simulink model "pharmacokinetics_model"  (R2022b)
settings: Solver=VariableStepAuto  StartTime=0.0  StopTime=total_time  RelTol=1e-3
values from neighbouring files (symbols this model uses):
  alpha = log(2)/half_life_bloodstream    [parameters.m]
  beta = log(2)/half_life_gi_tract    [parameters.m]
  initial_dosage = dosage_amount*60    (= 60000)    [parameters.m]
  pulse_period = 6    [parameters.m]
  pulse_width = ((1/pulse_period)/60)*100    (= 0.277777777778)    [parameters.m]
settings Model: Creator=wrickord  LastModifiedBy=wrick
settings ModelReferenceCC: EnableRefExpFcnMdlSchedulingChecks=on

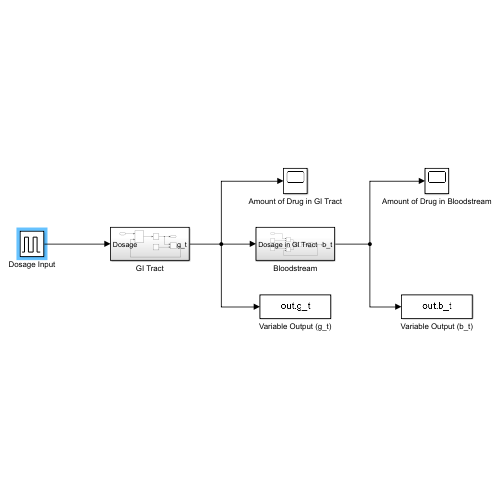
[thumbnail: Simulink's stored preview of the top-level diagram]
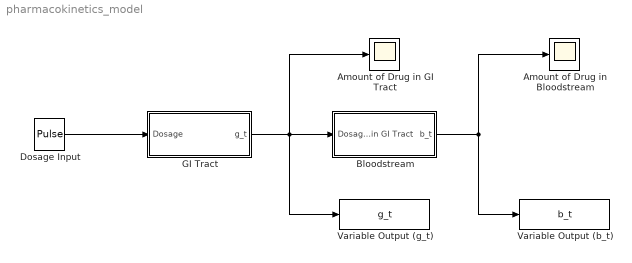
== system pharmacokinetics_model ==
  Amount of Drug in Bloodstream : Scope
  Amount of Drug in GI Tract : Scope
  Bloodstream : Subsystem
  Dosage Input : DiscretePulseGenerator  PulseType=Time based  Amplitude=initial_dosage  Period=pulse_period  PulseWidth=pulse_width
  GI Tract : Subsystem
  Variable Output (b_t) : ToWorkspace  VariableName=b_t  SampleTime=-1
  Variable Output (g_t) : ToWorkspace  VariableName=g_t  SampleTime=-1
  wires:
  GI Tract/1(g_t) -> Variable Output (g_t)/1, Amount of Drug in GI Tract/1, Bloodstream/1(Dosage in GI Tract)
  Bloodstream/1(b_t) -> Amount of Drug in Bloodstream/1, Variable Output (b_t)/1
  Dosage Input/1 -> GI Tract/1(Dosage)

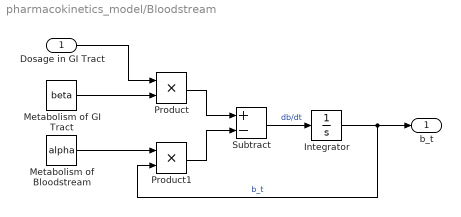
== system pharmacokinetics_model/Bloodstream ==
  Dosage in GI Tract : Inport
  Integrator : Integrator
  Metabolism of Bloodstream : Constant  Value=alpha
  Metabolism of GI Tract : Constant  Value=beta
  Product : Product
  Product1 : Product
  Subtract : Sum  Inputs=+-
  b_t : Outport
  wires:
  Metabolism of GI Tract/1 -> Product/2
  Dosage in GI Tract/1 -> Product/1
  Product/1 -> Subtract/1
  Product1/1 -> Subtract/2
  Subtract/1 -> Integrator/1  "db/dt"
  Metabolism of Bloodstream/1 -> Product1/1
  Integrator/1 -> b_t/1, Product1/2  "b_t"

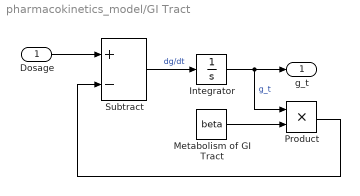
== system pharmacokinetics_model/GI Tract ==
  Dosage : Inport
  Integrator : Integrator
  Metabolism of GI Tract : Constant  Value=beta
  Product : Product
  Subtract : Sum  Inputs=+-
  g_t : Outport
  wires:
  Dosage/1 -> Subtract/1
  Product/1 -> Subtract/2
  Subtract/1 -> Integrator/1  "dg/dt"
  Integrator/1 -> g_t/1, Product/1  "g_t"
  Metabolism of GI Tract/1 -> Product/2
